simulink model "NarmaMotorNoDisrtubX"  (R2019b)
settings: Solver=FixedStepAuto  StartTime=0.0  StopTime=30  FixedStep=0.001  RelTol=1e-3
libraries: neural x1, simulink x1
settings Model: Creator=Emanuel  LastModifiedBy=Emanuel

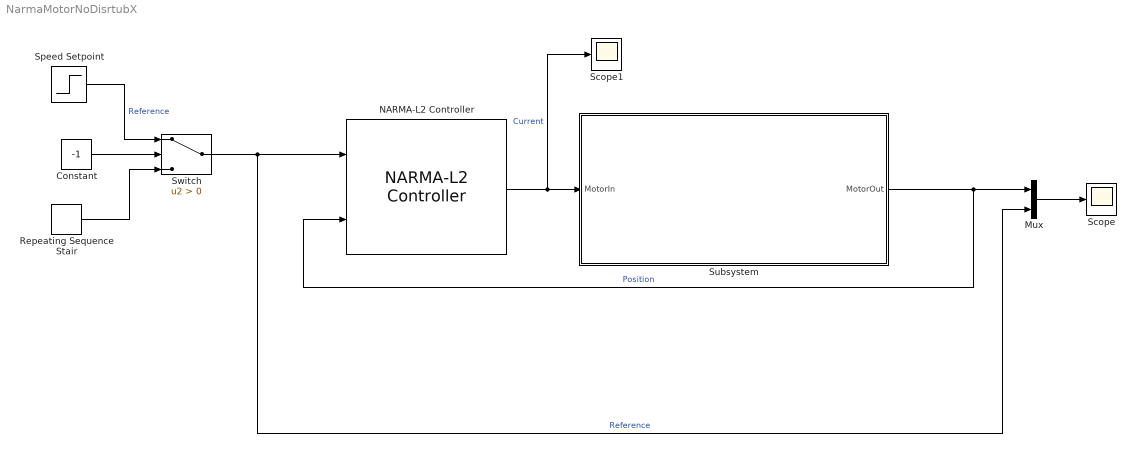
== system NarmaMotorNoDisrtubX ==
  Constant : Constant  Value=-1
  Mux : Mux  Inputs=2
  NARMA-L2 Controller : neural/Control Systems/NARMA-L2 Controller  Normalize=0  IW1_1=[6.3536413485183667049 1.2168838366603034196 -1.0269234832360636389 -2.2102308039093183645 -2.8958658472968665798 0.70007290105848662964 0.21805751202233900066 0.052509248970450048133 -0.075452401025514787003;9.2427343035550038053 9.2605127790416066347 9.3064361353107933894 9.3920465159864185978 9.5333874931160895727 0.027863322798428978577 0.013658530771708692064 0.060678041044878297527 -0.055391711609922393567;1.2162638402274592586 0.45755631319077511021 -0.36883906922289422248 -1.1684649052539415326 -1.8402540776802716049 0.049518260335746452916 0.10470432460013757991 0.10842770522565844948 0.10178292877326267085;1.7766676960654743667 -0.95965372923686642626 -0.21170798436150048416 0.82167379440516530309 1.5353457560426233552 0.3579660434822209969 -0.38331257765786785896 -0.46672859411925682327 -0.44409335532651672551;-0.00012302738462008718954 3.2610800000656975242e-05 -9.6134411118424021014e-06 -3.5485203650612109035e-06 1.3365600532569302077e-05 -0.00014596996571454324285 7.0654539563188119766e-05 8.7410135658881729691e-05 0.00017220210843266601955]  IW3_2=[0.093339296705841498514 -0.26192675798649445174 0.54222311287172408889 0.53855491793588350369 -0.66498177092394927801 -4.7419247342665071798 0.3037369196529854376 2.2328755337560060035 3.8188743787347014802;-0.17053480009835381148 0.55253726166084471405 -0.49532433901786648844 -0.10564183661598638975 0.26629404825103331067 -3.0252359181433914337 1.2259168218790790217 3.467933873588949556 2.4261966978204698719;-1.0788808043338100617 1.3890415003211760148 -0.44270730902599264578 0.4642841320746483591 -0.66034252984926822272 -2.7593457229500102379 2.0520275456500627342 3.3037503052783878665 4.2438002558187424285;-0.67495910859381225144 1.7734245748079517924 -0.99198975463519234452 -1.2296973757632556623 0.7988429647245743892 -2.3446170472084211234 0.043398572615602266922 -0.15936198548385033247 -1.1522254068279793593;-1.1301043518857030179 1.2454930019854719703 -0.20112788469465667229 1.0367605635876455672 -0.68004813196642321937 0.36573186610056207524 4.0838669875046145208 -1.4677517399202033577 3.2818966188396667683]  IW5_3=-1.0242506847954062632  LW2_1=[-12.176408697055450148 -12.039704214301282903 12.184118221247878466 -12.67968220768956833 104.11441181664326905]  LW4_3=[-0.27868116364863876333 2.3358114129653166913 -0.81122690924745788354 -1.5085391975395083808 1.399500544953939718]  LW5_4=1.4201278215305175312  LW6_5=-1.328800842557203099  LW6_2=-106.88485033752749587  B1=[-3.8052162230300190515;-0.58758577236639564223;-4.5551333306169334847;0.2452799067571395375;0.60062244588660240741]  B2=-12.471201640774692621  B3=[-4.8797284967633052233;-0.063261696781348283891;-1.7541329071681981411;-1.6046745050169846092;-0.59192977135025948154]  B4=-2.6205603891582844867  Limit_output=0  min_output=-Inf  max_output=Inf  Use_Previous_Weights=1  Ts=0.05  S1=5  Ni=5  Nj=5  sim_file=SoleModelNoDistrubance  trainfun=trainlm  Use_validation=1  Use_Testing=1  max_i=40  min_i=1  max_i_int=4  min_i_int=2  sam_training=10000  epochs=100  minp=1.2838861864609374397  maxp=39.753006491435613157  mint=2000.3866487334141766  maxt=39.753006491435613157
      settings: SourceProductName=Deep Learning Toolbox  SourceProductBaseCode=NN
  Repeating Sequence Stair : simulink/Sources/Repeating Sequence Stair  OutValues=[1000 2000 3000 4000 5000].'  tsamp=4  OutMin=[]  OutMax=[]  OutDataTypeStr=double  OutputDataTypeScalingMode=double  OutDataType=fixdt(0,8)  ConRadixGroup=Best Precision: Vector-wise  OutScaling=2^-12
  Scope : Scope
  Scope1 : Scope
  Speed Setpoint : Step  Time=5  Before=2000  After=3000  SampleTime=0
  Subsystem : Subsystem
  Switch : Switch  Criteria=u2 > Threshold
  wires:
  NARMA-L2 Controller/1 -> Scope1/1, Subsystem/1(MotorIn)  "Current"
  Subsystem/1("MotorOut ") -> NARMA-L2 Controller/2, Mux/1  "Position"
  Mux/1 -> Scope/1
  Switch/1 -> Mux/2, NARMA-L2 Controller/1  "Reference"
  Repeating Sequence Stair/1 -> Switch/3
  Speed Setpoint/1 -> Switch/1  "Reference"
  Constant/1 -> Switch/2

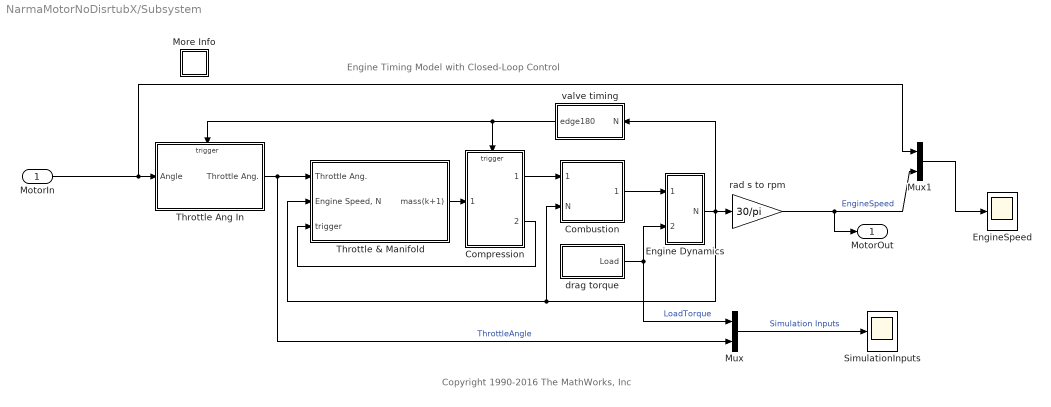
== system NarmaMotorNoDisrtubX/Subsystem ==
  note: Copyright 1990-2016 The MathWorks, Inc
  note: Engine Timing Model with Closed-Loop Control
  MotorIn : Inport
  Combustion : Subsystem
  Compression : Subsystem  TreatAsAtomicUnit=on
  Engine Dynamics : Subsystem
  EngineSpeed : Scope
  More Info : Subsystem
      settings: OpenFcn=showdemo(bdroot(gcb))
      mask Display: disp('?')
  Mux : Mux  Inputs=2
  Mux1 : Mux  Inputs=2
  SimulationInputs : Scope
  Throttle & Manifold : Subsystem
  Throttle Ang In : Subsystem  TreatAsAtomicUnit=on
  drag torque : Subsystem
  rad s to rpm : Gain  Gain=30/pi  SaturateOnIntegerOverflow=on  OutDataTypeStr=Inherit: Same as input  ParamDataTypeStr=Inherit: Same as input
  valve timing : Subsystem
  "MotorOut " : Outport
  wires:
  Combustion/1(Torque) -> Engine Dynamics/1(Teng)
  Throttle Ang In/1(Throttle Ang.) -> Mux/2, Throttle & Manifold/1(Throttle Ang.)  "ThrottleAngle"
  drag torque/1(Load) -> Mux/1, Engine Dynamics/2(Tload)  "LoadTorque"
  MotorIn/1 -> Mux1/1, Throttle Ang In/1(Angle)
  Throttle & Manifold/1(mass(k+1)) -> Compression/1(mass(k+1))
  Compression/2(trigger) -> Throttle & Manifold/3(trigger)
  Mux/1 -> SimulationInputs/1  "Simulation Inputs"
  rad s to rpm/1 -> "MotorOut "/1, Mux1/2  "EngineSpeed"
  Compression/1(mass(k)) -> Combustion/1(Air Charge)
  Mux1/1 -> EngineSpeed/1
  valve timing/1(edge180) -> Throttle Ang In/Trigger, Compression/Trigger
  Engine Dynamics/1(N) -> rad s to rpm/1, valve timing/1(N), Throttle & Manifold/2("Engine Speed, N"), Combustion/2(N)

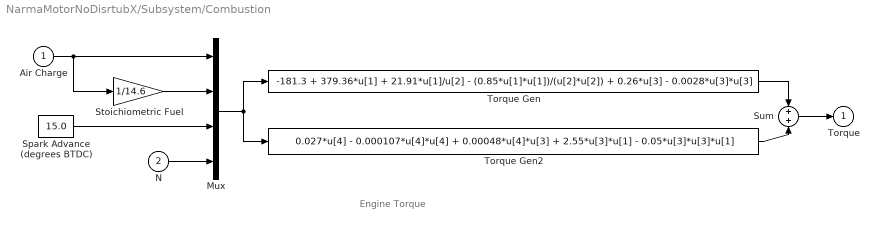
== system NarmaMotorNoDisrtubX/Subsystem/Combustion ==
  note: Engine Torque
  Air Charge : Inport
  N : Inport  Port=2
  Mux : Mux
  Spark Advance (degrees BTDC) : Constant  Value=15.0
  Stoichiometric Fuel : Gain  Gain=1/14.6  SaturateOnIntegerOverflow=on  OutDataTypeStr=Inherit: Same as input  ParamDataTypeStr=Inherit: Same as input
  Sum : Sum  SaturateOnIntegerOverflow=on  InputSameDT=on  OutDataTypeStr=Inherit: Same as first input
  Torque Gen : Fcn  Expr=-181.3 + 379.36*u[1] + 21.91*u[1]/u[2] - (0.85*u[1]*u[1])/(u[2]*u[2]) + 0.26*u[3] - 0.0028*u[3]*u[3]
  Torque Gen2 : Fcn  Expr=0.027*u[4] - 0.000107*u[4]*u[4] + 0.00048*u[4]*u[3] + 2.55*u[3]*u[1] - 0.05*u[3]*u[3]*u[1]
  Torque : Outport  InitialOutput=0
  wires:
  Stoichiometric Fuel/1 -> Mux/2
  Spark Advance (degrees BTDC)/1 -> Mux/3
  N/1 -> Mux/4
  Air Charge/1 -> Stoichiometric Fuel/1, Mux/1
  Mux/1 -> Torque Gen/1, Torque Gen2/1
  Torque Gen2/1 -> Sum/2
  Torque Gen/1 -> Sum/1
  Sum/1 -> Torque/1

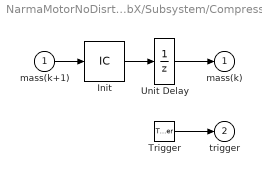
== system NarmaMotorNoDisrtubX/Subsystem/Compression ==
  mass(k+1) : Inport
  Trigger : TriggerPort  TriggerType=either  VariantControl=Variant  ShowOutputPort=on
  Init : InitialCondition  Value=0.152
  Unit Delay : UnitDelay  InitialCondition=0.152  SampleTime=-1  HasFrameUpgradeWarning=on
  mass(k) : Outport  InitialOutput=0.152
  trigger : Outport  Port=2  InitialOutput=-1
  wires:
  Init/1 -> Unit Delay/1
  mass(k+1)/1 -> Init/1
  Unit Delay/1 -> mass(k)/1
  Trigger/1 -> trigger/1

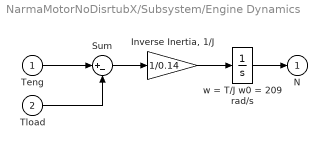
== system NarmaMotorNoDisrtubX/Subsystem/Engine Dynamics ==
  Teng : Inport
  Tload : Inport  Port=2
  "Inverse Inertia, 1/J" : Gain  Gain=1/0.14  SaturateOnIntegerOverflow=on  OutDataTypeStr=Inherit: Same as input  ParamDataTypeStr=Inherit: Same as input
  Sum : Sum  Inputs=|+-  SaturateOnIntegerOverflow=on  InputSameDT=on  OutDataTypeStr=Inherit: Same as first input
  w = T/J w0 = 209 rad/s : Integrator  InitialCondition=209.48
  N : Outport  InitialOutput=0
  wires:
  "Inverse Inertia, 1/J"/1 -> w = T/J w0 = 209 rad/s/1
  w = T/J w0 = 209 rad/s/1 -> N/1
  Sum/1 -> "Inverse Inertia, 1/J"/1
  Teng/1 -> Sum/1
  Tload/1 -> Sum/2

== system NarmaMotorNoDisrtubX/Subsystem/More Info ==

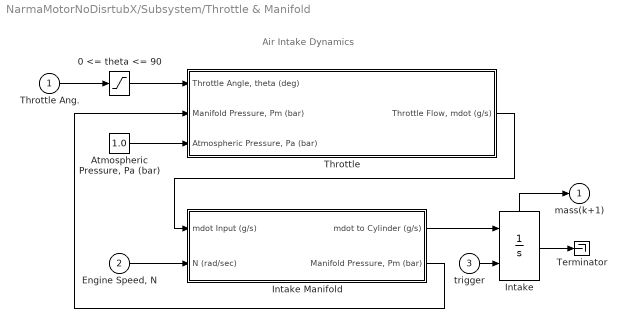
== system NarmaMotorNoDisrtubX/Subsystem/Throttle & Manifold ==
  note: Air Intake Dynamics
  Throttle Ang. : Inport
  "Engine Speed, N" : Inport  Port=2
  trigger : Inport  Port=3
  0 <= theta <= 90 : Saturate  UpperLimit=90  LowerLimit=0
  "Atmospheric Pressure, Pa (bar)" : Constant  Value=1.0
  Intake : Integrator  ExternalReset=either  ShowStatePort=on
  Intake Manifold : Subsystem
  Terminator : Terminator
  Throttle : Subsystem
  mass(k+1) : Outport  InitialOutput=0
  wires:
  0 <= theta <= 90/1 -> Throttle/1("Throttle Angle, theta (deg)")
  Throttle Ang./1 -> 0 <= theta <= 90/1
  Throttle/1("Throttle Flow, mdot (g/s)") -> Intake Manifold/1(mdot Input (g/s))
  "Engine Speed, N"/1 -> Intake Manifold/2(N (rad/sec))
  Intake Manifold/2("Manifold Pressure, Pm (bar)") -> Throttle/2("Manifold Pressure, Pm (bar)")
  Intake Manifold/1(mdot to Cylinder (g/s)) -> Intake/1
  "Atmospheric Pressure, Pa (bar)"/1 -> Throttle/3("Atmospheric Pressure, Pa (bar) ")
  Intake/State -> mass(k+1)/1
  trigger/1 -> Intake/2
  Intake/1 -> Terminator/1

== system NarmaMotorNoDisrtubX/Subsystem/Throttle Ang In ==
  note: Controller Subsystem
  Angle : Inport
  Trigger : TriggerPort  TriggerType=either  VariantControl=Variant
  Throttle Ang. : Outport  InitialOutput=8.973
  wires:
  Angle/1 -> Throttle Ang./1

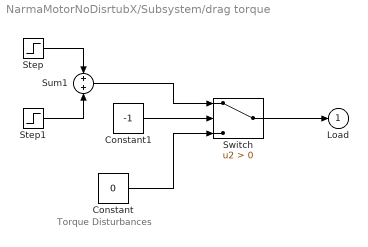
== system NarmaMotorNoDisrtubX/Subsystem/drag torque ==
  note: Torque Disturbances
  Constant : Constant  Value=0
  Constant1 : Constant  Value=-1
  Step : Step  Time=2  Before=25  After=20  SampleTime=0
  Step1 : Step  Time=8  After=5  SampleTime=0
  Sum1 : Sum  SaturateOnIntegerOverflow=on  InputSameDT=on  OutDataTypeStr=Inherit: Same as first input
  Switch : Switch  Criteria=u2 > Threshold
  Load : Outport  InitialOutput=0
  wires:
  Sum1/1 -> Switch/1
  Step/1 -> Sum1/1
  Step1/1 -> Sum1/2
  Switch/1 -> Load/1
  Constant/1 -> Switch/3
  Constant1/1 -> Switch/2

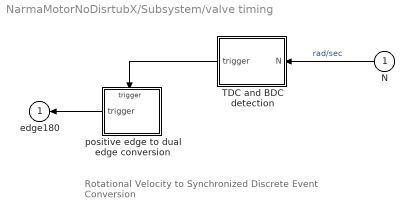
== system NarmaMotorNoDisrtubX/Subsystem/valve timing ==
  note: Rotational Velocity to Synchronized
      | Discrete Event Conversion
  N : Inport
  TDC and BDC detection : Subsystem
  positive edge to dual edge conversion : Subsystem  TreatAsAtomicUnit=on
  edge180 : Outport  InitialOutput=-1
  wires:
  TDC and BDC detection/1(trigger) -> positive edge to dual edge conversion/Trigger
  positive edge to dual edge conversion/1(trigger) -> edge180/1
  N/1 -> TDC and BDC detection/1(N)  "rad/sec"

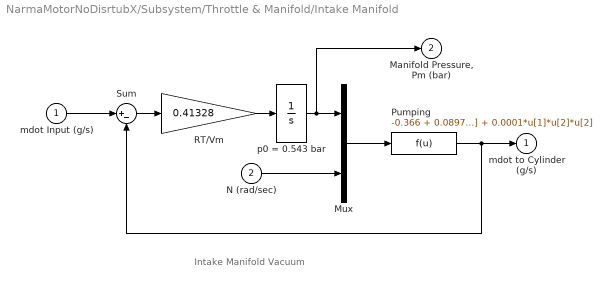
== system NarmaMotorNoDisrtubX/Subsystem/Throttle & Manifold/Intake Manifold ==
  note: Intake Manifold Vacuum
  mdot Input (g/s) : Inport
  N (rad/sec) : Inport  Port=2
  Mux : Mux  Inputs=2
  Pumping : Fcn  Expr=-0.366 + 0.08979*u[1]*u[2] - 0.0337*u[2]*u[1]*u[1] + 0.0001*u[1]*u[2]*u[2]
  RT/Vm : Gain  Gain=0.41328  SaturateOnIntegerOverflow=on  OutDataTypeStr=Inherit: Same as input  ParamDataTypeStr=Inherit: Same as input
  Sum : Sum  Inputs=|+-  SaturateOnIntegerOverflow=on  InputSameDT=on  OutDataTypeStr=Inherit: Same as first input
  p0 = 0.543 bar : Integrator  InitialCondition=.543
  mdot to Cylinder (g/s) : Outport  InitialOutput=0
  "Manifold Pressure, Pm (bar)" : Outport  Port=2  InitialOutput=0
  wires:
  mdot Input (g/s)/1 -> Sum/1
  RT/Vm/1 -> p0 = 0.543 bar/1
  N (rad/sec)/1 -> Mux/2
  Mux/1 -> Pumping/1
  p0 = 0.543 bar/1 -> Mux/1, "Manifold Pressure, Pm (bar)"/1
  Sum/1 -> RT/Vm/1
  Pumping/1 -> Sum/2, mdot to Cylinder (g/s)/1

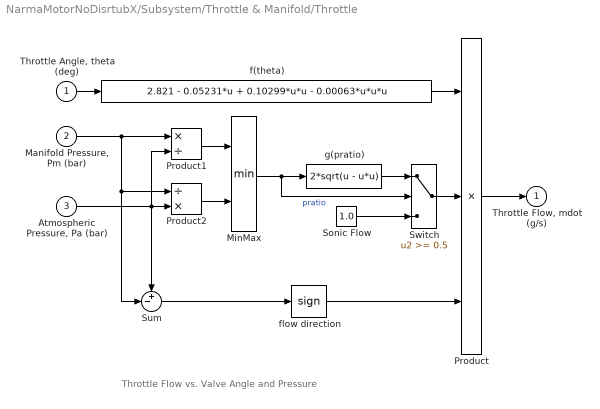
== system NarmaMotorNoDisrtubX/Subsystem/Throttle & Manifold/Throttle ==
  note: Throttle Flow vs. Valve Angle and Pressure
  "Throttle Angle, theta (deg)" : Inport
  "Manifold Pressure, Pm (bar)" : Inport  Port=2
  "Atmospheric Pressure, Pa (bar) " : Inport  Port=3
  MinMax : MinMax  Inputs=2  SaturateOnIntegerOverflow=on  InputSameDT=on
  Product : Product  Inputs=3  SaturateOnIntegerOverflow=on  RndMeth=Zero  InputSameDT=on  OutDataTypeStr=Inherit: Same as first input
  Product1 : Product  Inputs=*/  SaturateOnIntegerOverflow=on  RndMeth=Zero  InputSameDT=on  OutDataTypeStr=Inherit: Same as first input
  Product2 : Product  Inputs=/*  SaturateOnIntegerOverflow=on  RndMeth=Zero  InputSameDT=on  OutDataTypeStr=Inherit: Same as first input
  "Sonic Flow " : Constant  Value=1.0
  Sum : Sum  Inputs=+-|  SaturateOnIntegerOverflow=on  InputSameDT=on  OutDataTypeStr=Inherit: Same as first input
  Switch : Switch  Threshold=0.5  SaturateOnIntegerOverflow=on  InputSameDT=on
  f(theta) : Fcn  Expr=2.821 - 0.05231*u + 0.10299*u*u - 0.00063*u*u*u
  flow direction : Signum
  g(pratio) : Fcn  Expr=2*sqrt(u - u*u)
  "Throttle Flow, mdot (g/s)" : Outport  InitialOutput=0
  wires:
  "Manifold Pressure, Pm (bar)"/1 -> Sum/2, Product2/1, Product1/1
  Product2/1 -> MinMax/2
  Product1/1 -> MinMax/1
  "Atmospheric Pressure, Pa (bar) "/1 -> Sum/1, Product2/2, Product1/2
  g(pratio)/1 -> Switch/1
  "Sonic Flow "/1 -> Switch/3
  Switch/1 -> Product/2
  flow direction/1 -> Product/3
  Sum/1 -> flow direction/1
  MinMax/1 -> Switch/2, g(pratio)/1  "pratio"
  "Throttle Angle, theta (deg)"/1 -> f(theta)/1
  Product/1 -> "Throttle Flow, mdot (g/s)"/1
  f(theta)/1 -> Product/1

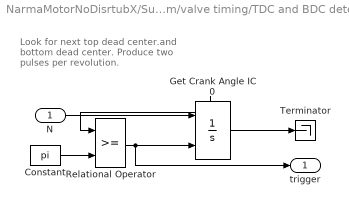
== system NarmaMotorNoDisrtubX/Subsystem/valve timing/TDC and BDC detection ==
  note: Look for next top dead center.and
      | bottom dead center.
      | Produce two pulses per revolution.
  N : Inport
  Constant : Constant  Value=pi
  Get Crank Angle IC 0 : Integrator  ExternalReset=rising  ShowStatePort=on
  Relational Operator : RelationalOperator  OutDataTypeStr=boolean  RndMeth=Nearest  InputSameDT=on
  Terminator : Terminator
  trigger : Outport  InitialOutput=0
  wires:
  N/1 -> Get Crank Angle IC 0/1
  Relational Operator/1 -> trigger/1, Get Crank Angle IC 0/2
  Constant/1 -> Relational Operator/2
  Get Crank Angle IC 0/State -> Relational Operator/1
  Get Crank Angle IC 0/1 -> Terminator/1

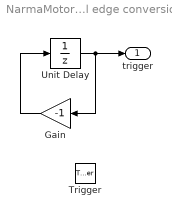
== system NarmaMotorNoDisrtubX/Subsystem/valve timing/positive edge to dual edge conversion ==
  Trigger : TriggerPort  VariantControl=Variant
  Gain : Gain  Gain=-1  SaturateOnIntegerOverflow=on  OutDataTypeStr=Inherit: Same as input  ParamDataTypeStr=Inherit: Same as input
  Unit Delay : UnitDelay  InitialCondition=1  SampleTime=-1  HasFrameUpgradeWarning=on
  trigger : Outport  InitialOutput=-1
  wires:
  Gain/1 -> Unit Delay/1
  Unit Delay/1 -> trigger/1, Gain/1
